simulink subsystem "subsistema_termico"  (R2023b)
settings: Solver=VariableStepAuto  StartTime=0.0  StopTime=10.0  RelTol=1e-3
values from neighbouring files (symbols this model uses):
  alpha_cu = 3.9 * 10^(-3)    (= 0.0039)    [parametros.m]
  C_ts = 0.818    [parametros.m]
  R_sref = 1.02    [parametros.m]
  R_tsamb = 146.7    [parametros.m]
  T_sref = 20    [parametros.m]
settings Model: Creator=nicol  LastModifiedBy=Julya

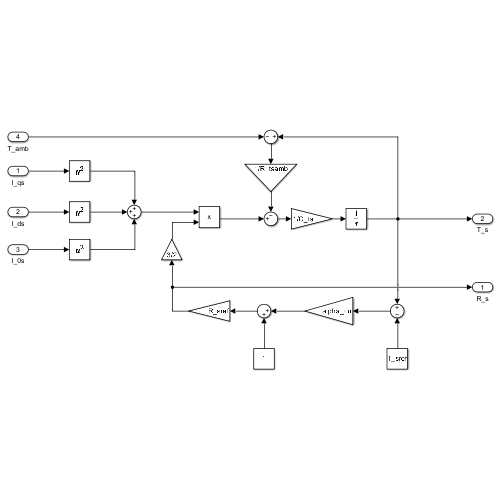
[thumbnail: Simulink's stored preview of the top-level diagram]
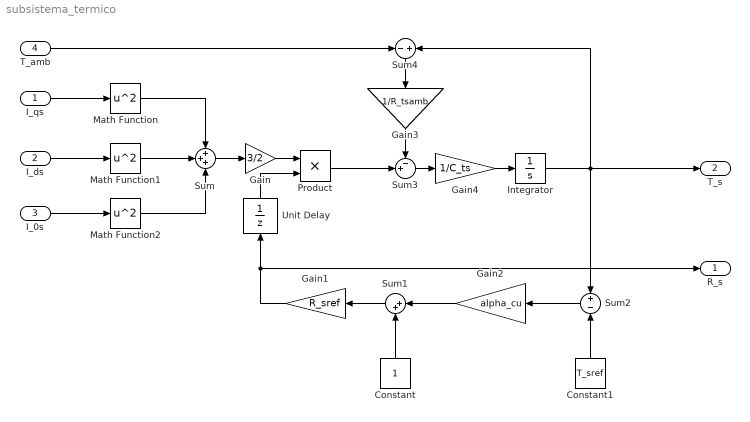
== system subsistema_termico ==
  I_qs : Inport
  I_ds : Inport  Port=2
  I_0s : Inport  Port=3
  T_amb : Inport  Port=4
  Constant : Constant
  Constant1 : Constant  Value=T_sref
  Gain : Gain  Gain=3/2
  Gain1 : Gain  Gain=R_sref
  Gain2 : Gain  Gain=alpha_cu
  Gain3 : Gain  Gain=1/R_tsamb
  Gain4 : Gain  Gain=1/C_ts
  Integrator : Integrator  InitialCondition=20
  Math Function : Math  Operator=square
  Math Function1 : Math  Operator=square
  Math Function2 : Math  Operator=square
  Product : Product
  Sum : Sum  Inputs=+++
  Sum1 : Sum  Inputs=|++
  Sum2 : Sum  Inputs=+|-
  Sum3 : Sum  Inputs=-+|
  Sum4 : Sum  Inputs=-|+
  Unit Delay : UnitDelay  SampleTime=1e-5  HasFrameUpgradeWarning=on
  R_s : Outport
  T_s : Outport  Port=2
  wires:
  Math Function2/1 -> Sum/3
  Math Function1/1 -> Sum/2
  Math Function/1 -> Sum/1
  I_ds/1 -> Math Function1/1
  I_0s/1 -> Math Function2/1
  I_qs/1 -> Math Function/1
  Gain1/1 -> Unit Delay/1, R_s/1
  Sum/1 -> Gain/1
  Sum1/1 -> Gain1/1
  Constant/1 -> Sum1/2
  Constant1/1 -> Sum2/2
  Gain2/1 -> Sum1/1
  Sum2/1 -> Gain2/1
  T_amb/1 -> Sum4/1
  Sum4/1 -> Gain3/1
  Gain3/1 -> Sum3/1
  Product/1 -> Sum3/2
  Gain4/1 -> Integrator/1
  Sum3/1 -> Gain4/1
  Integrator/1 -> Sum4/2, T_s/1, Sum2/1
  Gain/1 -> Product/1
  Unit Delay/1 -> Product/2
